simulink model "Identif_OpenLoop"  (R2023b)
settings: Solver=VariableStepAuto  StartTime=0.0  StopTime=80  FixedStep=0.0001  RelTol=1e-3
values from neighbouring files (symbols this model uses):
  C_T = Tg_ss / (r_r^4 * rho_air * pi * w_ss^2 * L_rod)    (= 0.0178337228008)    [model_constants.m]
  g = 9.81    [ArisonaIden.m]    (also in may13.m; model_constants.m = 9.806)
  J = 0.048    [ArisonaIden.m]    (also in may13.m; model_constants.m = 0.0161112)
  K_bldc = 131.3016804    [model_constants.m]
  K_f1 = r_r^4 * rho_air * pi * C_T    (= 5.49430535846e-06)    [model_constants.m]
  K_f2 = K_f1 * w_ss^2 / u_ss    (= 0.327888125)    [model_constants.m]
  L_g = (m_mot*L_rod + m_rod*L_rod/2)/(m_rod + m_mot)    (= 0.291818181818)    [model_constants.m]
  L_rod = 0.57    [ArisonaIden.m]    (also in model_constants.m = 0.42)
  m_mot = 0.06    [model_constants.m]
  m_rod = m_esc + m_ardu + m_wood    (= 0.094)    [model_constants.m]
  r_r = 0.095    [model_constants.m]
  rho_air = 1.204    [model_constants.m]
  Sample_Time = 0.025 * 2    (= 0.05)    [model_constants.m]
  T_bldc = 0.010214509    [model_constants.m]
undefined symbols (not defined in the file or in its folder): LF
libraries: slpidlib x8, instrumentseriallib x3, sldrtlib x2, svdutilitieslib x1
settings Model: SimulationMode=accelerator  Creator=Илья  LastModifiedBy=Илья

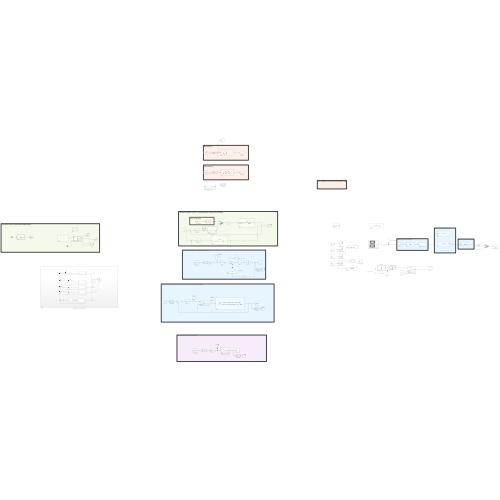
[thumbnail: Simulink's stored preview of the top-level diagram]
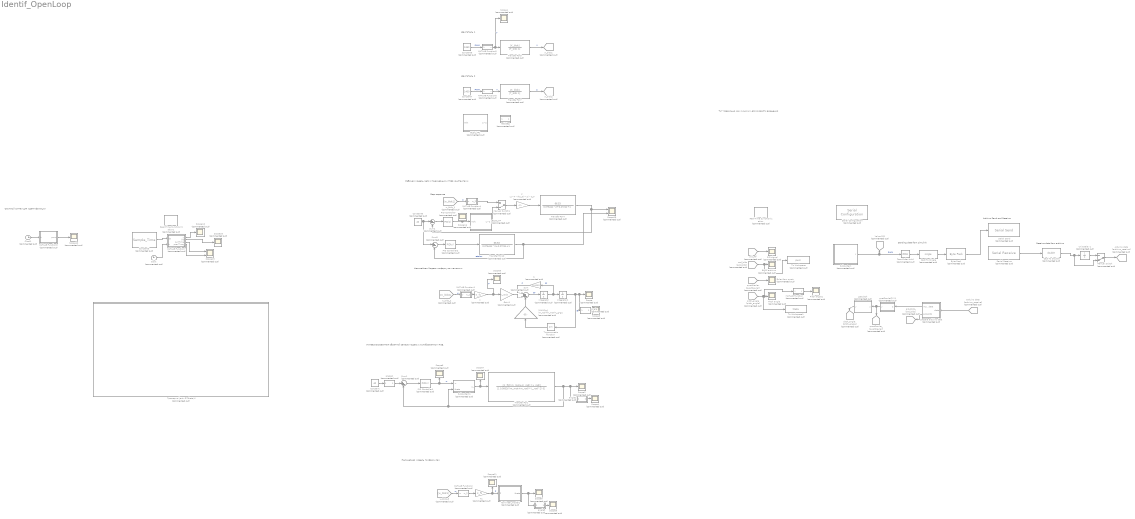
== system Identif_OpenLoop ==
  note: Нелинейная Модель из формулы механики
  note: Тут правильно как минимум для скорости вращения
  note: Sending data from simulink
  note: Arduino Send and Receive
  note: Receive data from arduino
  note: Step response
  note: Двигатель 1
  note: Двигатель 2
  note: Рабочая модель ijertv с подходящими ПИД константами
  note: Линеаризированная обратной связью модель с колиброванным ПИД
  note: Сложный сигнал для идентификации
  note: Нелинейная модель по формулам
  (M+M)lg/J : Gain  Commented=on  Gain=(m_rod+m_mot)*L_g*g/J
  Arduino data : Goto  Commented=on  GotoTag=arduino_receive
  BLDC arduino : Scope  Commented=on
  BLDC_TF : Subsystem  Commented=on
  BLDC_TF1 : Subsystem  Commented=on
  Byte Pack : svdutilitieslib/Byte Pack  Commented=on  maskPackedDataType=uint32  datatypes={'single'}  byteAlign=4  blockPlatform=arduinoert
  Cast To Double : DataTypeConversion  Commented=on  OutDataTypeStr=double  SaturateOnIntegerOverflow=off  RndMeth=Floor
  Cast To Single : DataTypeConversion  Commented=on  OutDataTypeStr=single  SaturateOnIntegerOverflow=off  RndMeth=Floor
  Clock : Clock  Commented=on
  Clock1 : Clock  Commented=on
  Constant : Constant  Commented=on  Value=40
  Constant3 : Constant  Commented=on  Value=Sample_Time
  Constant5 : Constant  Commented=on  Value=1350
  Constant6 : Constant  Commented=on  Value=40
  Constant7 : Constant  Commented=on  Value=1400
  Euler from quart : Scope  Commented=on
  F : Gain  Commented=on  Gain=r_r^4 * rho_air * pi * C_T
  Gain1 : Gain  Commented=on  Gain=L_rod/J
  Integrator : Integrator  Commented=on
  Integrator1 : Integrator  Commented=on
  K : Gain  Commented=on  Gain=K_f1
  K1 : Gain  Commented=on  Gain=K_f1
  MATLAB Function : MATLAB Function  Commented=on  TreatAsAtomicUnit=on
  MATLAB Function1 : MATLAB Function  Commented=on  TreatAsAtomicUnit=on
  MATLAB Function2 : MATLAB Function  Commented=on  TreatAsAtomicUnit=on
  MATLAB Function3 : MATLAB Function  Commented=on  TreatAsAtomicUnit=on
  MATLAB Function4 : MATLAB Function  Commented=on  TreatAsAtomicUnit=on
  MATLAB Function5 : MATLAB Function  Commented=on  TreatAsAtomicUnit=on
  MATLAB Function6 : MATLAB Function  Commented=on  TreatAsAtomicUnit=on
  MATLAB Function7 : MATLAB Function  Commented=on  TreatAsAtomicUnit=on  SystemSampleTime=Sample_Time
  Manual Switch : ManualSwitch  Commented=on  CurrentSetting=0
  Manual Switch1 : ManualSwitch  Commented=on  CurrentSetting=0
  Nonlinear_model1 : Subsystem  Commented=on
  PID Controller : slpidlib/PID Controller  Commented=on  Controller=PID  Form=Parallel  TimeDomain=Continuous-time  UseExternalTs=off  SampleTime=-1  IntegratorMethod=Forward Euler  FilterMethod=Forward Euler  ControllerParametersSource=internal  P=0.00834  I=0.0329  UseKiTs=off  D=0.00053  N=100  UseFilter=on  TunerSelectOption=Transfer Function Based (PID Tuner App)  InitialConditionSource=internal  InitialConditionForIntegrator=0  InitialConditionForFilter=0  DifferentiatorICPrevScaledInput=0  ExternalReset=none  TrackingMode=off  Kt=1  LimitOutput=off  SatLimitsSource=internal  UpperSaturationLimit=inf  LowerSaturationLimit=-inf  LinearizeAsGain=on  AntiWindupMode=none  Kb=1  LimitIntegrator=off  UpperIntegratorSaturationLimit=inf  LowerIntegratorSaturationLimit=-inf  POutMin=[]  POutMax=[]  IOutMin=[]  IOutMax=[]  DOutMin=[]  DOutMax=[]  NOutMin=[]  NOutMax=[]  SumOutMin=[]  SumOutMax=[]  SaturationOutMin=[]  SaturationOutMax=[]  PParamMin=[]  PParamMax=[]  IParamMin=[]  IParamMax=[]  DParamMin=[]  DParamMax=[]  NParamMin=[]  NParamMax=[]  KbParamMin=[]  KbParamMax=[]  KtParamMin=[]  KtParamMax=[]  KbOutMin=[]  KbOutMax=[]  KtOutMin=[]  KtOutMax=[]  IntegratorOutMin=[]  IntegratorOutMax=[]  FilterOutMin=[]  FilterOutMax=[]  SumI1OutMin=[]  SumI1OutMax=[]  SumI2OutMin=[]  SumI2OutMax=[]  SumI3OutMin=[]  SumI3OutMax=[]  SumI4OutMin=[]  SumI4OutMax=[]  SumDOutMin=[]  SumDOutMax=[]  DifferentiatorOutMin=[]  DifferentiatorOutMax=[]  FilterDiffOutCoefMin=[]  FilterDiffOutCoefMax=[]  ReciprocalOutMin=[]  ReciprocalOutMax=[]  SumDenOutMin=[]  SumDenOutMax=[]  SumNumOutMin=[]  SumNumOutMax=[]  DivideOutMin=[]  DivideOutMax=[]  UdiffTsProdOutMin=[]  UdiffTsProdOutMax=[]  NTsProdOutMin=[]  NTsProdOutMax=[]  UintegralTsProdOutMin=[]  UintegralTsProdOutMax=[]  UngainTsProdOutMin=[]  UngainTsProdOutMax=[]  ClampingZeroOutDataTypeStr=Inherit: Inherit via back propagation  ClampingZeroOutMin=[]  ClampingZeroOutMax=[]  FilterDenConstantOutDataTypeStr=Inherit: Inherit via back propagation  FilterDenConstantOutMin=[]  FilterDenConstantOutMax=[]  PCopyOutDataTypeStr=Inherit: Inherit via back propagation  PCopyOutMin=[]  PCopyOutMax=[]  NCopyOutDataTypeStr=Inherit: Inherit via back propagation  NCopyOutMin=[]  NCopyOutMax=[]  IntegratorContinuousStateAttributes=''  IntegratorStateMustResolveToSignalObject=off  IntegratorRTWStateStorageClass=Auto  FilterContinuousStateAttributes=''  FilterStateMustResolveToSignalObject=off  FilterRTWStateStorageClass=Auto  ParallelPVariant=InternalParameters  IdealPVariant=Disabled  IVariant=InternalParameters  DVariant=InternalParameters  IntegratorVariant=Continuous  SatVariant=Disabled  AWVariant=Passthrough  PCopyVariant=Disabled  TRVariant=Disabled  FdbkBlocksVariant=Forward  IdealPFdbkVariant=Disabled  SatFdbkVariant=Disabled  DerivativeFilterVariant=ContFilter  NVariant=InternalParameters  NCopyVariant=Disabled  FilterICVariant=InternalICsFilter  IntegratorICVariant=InternalICs  ExternalResetVariant=Disabled  TRSumVariant=Passthrough  SumFdbkVariant=Disabled  SumVariant=Sum_PID  TsampFilterVariant=InternalTs  TsampNgainVariant=Passthrough  TsampIntegralVariant=Disabled_SignalSpec  ExternalSaturationOutDataTypeStr=Inherit: Same as second input
  PID Controller1 : slpidlib/PID Controller  Commented=on  Controller=PID  Form=Parallel  TimeDomain=Continuous-time  UseExternalTs=off  SampleTime=-1  IntegratorMethod=Forward Euler  FilterMethod=Forward Euler  ControllerParametersSource=internal  P=822.969764124437  I=5665.62260200918  UseKiTs=off  D=29.2943119385291  N=827.781411873675  UseFilter=on  TunerSelectOption=Transfer Function Based (PID Tuner App)  InitialConditionSource=internal  InitialConditionForIntegrator=0  InitialConditionForFilter=0  DifferentiatorICPrevScaledInput=0  ExternalReset=none  TrackingMode=off  Kt=1  LimitOutput=off  SatLimitsSource=internal  UpperSaturationLimit=inf  LowerSaturationLimit=-inf  LinearizeAsGain=on  AntiWindupMode=none  Kb=1  LimitIntegrator=off  UpperIntegratorSaturationLimit=inf  LowerIntegratorSaturationLimit=-inf  POutMin=[]  POutMax=[]  IOutMin=[]  IOutMax=[]  DOutMin=[]  DOutMax=[]  NOutMin=[]  NOutMax=[]  SumOutMin=[]  SumOutMax=[]  SaturationOutMin=[]  SaturationOutMax=[]  PParamMin=[]  PParamMax=[]  IParamMin=[]  IParamMax=[]  DParamMin=[]  DParamMax=[]  NParamMin=[]  NParamMax=[]  KbParamMin=[]  KbParamMax=[]  KtParamMin=[]  KtParamMax=[]  KbOutMin=[]  KbOutMax=[]  KtOutMin=[]  KtOutMax=[]  IntegratorOutMin=[]  IntegratorOutMax=[]  FilterOutMin=[]  FilterOutMax=[]  SumI1OutMin=[]  SumI1OutMax=[]  SumI2OutMin=[]  SumI2OutMax=[]  SumI3OutMin=[]  SumI3OutMax=[]  SumI4OutMin=[]  SumI4OutMax=[]  SumDOutMin=[]  SumDOutMax=[]  DifferentiatorOutMin=[]  DifferentiatorOutMax=[]  FilterDiffOutCoefMin=[]  FilterDiffOutCoefMax=[]  ReciprocalOutMin=[]  ReciprocalOutMax=[]  SumDenOutMin=[]  SumDenOutMax=[]  SumNumOutMin=[]  SumNumOutMax=[]  DivideOutMin=[]  DivideOutMax=[]  UdiffTsProdOutMin=[]  UdiffTsProdOutMax=[]  NTsProdOutMin=[]  NTsProdOutMax=[]  UintegralTsProdOutMin=[]  UintegralTsProdOutMax=[]  UngainTsProdOutMin=[]  UngainTsProdOutMax=[]  ClampingZeroOutDataTypeStr=Inherit: Inherit via back propagation  ClampingZeroOutMin=[]  ClampingZeroOutMax=[]  FilterDenConstantOutDataTypeStr=Inherit: Inherit via back propagation  FilterDenConstantOutMin=[]  FilterDenConstantOutMax=[]  PCopyOutDataTypeStr=Inherit: Inherit via back propagation  PCopyOutMin=[]  PCopyOutMax=[]  NCopyOutDataTypeStr=Inherit: Inherit via back propagation  NCopyOutMin=[]  NCopyOutMax=[]  IntegratorContinuousStateAttributes=''  IntegratorStateMustResolveToSignalObject=off  IntegratorRTWStateStorageClass=Auto  FilterContinuousStateAttributes=''  FilterStateMustResolveToSignalObject=off  FilterRTWStateStorageClass=Auto  ParallelPVariant=InternalParameters  IdealPVariant=Disabled  IVariant=InternalParameters  DVariant=InternalParameters  IntegratorVariant=Continuous  SatVariant=Disabled  AWVariant=Passthrough  PCopyVariant=Disabled  TRVariant=Disabled  FdbkBlocksVariant=Forward  IdealPFdbkVariant=Disabled  SatFdbkVariant=Disabled  DerivativeFilterVariant=ContFilter  NVariant=InternalParameters  NCopyVariant=Disabled  FilterICVariant=InternalICsFilter  IntegratorICVariant=InternalICs  ExternalResetVariant=Disabled  TRSumVariant=Passthrough  SumFdbkVariant=Disabled  SumVariant=Sum_PID  TsampFilterVariant=InternalTs  TsampNgainVariant=Passthrough  TsampIntegralVariant=Disabled_SignalSpec  ExternalSaturationOutDataTypeStr=Inherit: Same as second input
  PID Controller2 : slpidlib/PID Controller  Commented=on  Controller=PID  Form=Parallel  TimeDomain=Continuous-time  UseExternalTs=off  SampleTime=-1  IntegratorMethod=Forward Euler  FilterMethod=Forward Euler  ControllerParametersSource=internal  P=0.00834  I=0.0329  UseKiTs=off  D=0.00053  N=100  UseFilter=on  TunerSelectOption=Transfer Function Based (PID Tuner App)  InitialConditionSource=internal  InitialConditionForIntegrator=0  InitialConditionForFilter=0  DifferentiatorICPrevScaledInput=0  ExternalReset=none  TrackingMode=off  Kt=1  LimitOutput=off  SatLimitsSource=internal  UpperSaturationLimit=inf  LowerSaturationLimit=-inf  LinearizeAsGain=on  AntiWindupMode=none  Kb=1  LimitIntegrator=off  UpperIntegratorSaturationLimit=inf  LowerIntegratorSaturationLimit=-inf  POutMin=[]  POutMax=[]  IOutMin=[]  IOutMax=[]  DOutMin=[]  DOutMax=[]  NOutMin=[]  NOutMax=[]  SumOutMin=[]  SumOutMax=[]  SaturationOutMin=[]  SaturationOutMax=[]  PParamMin=[]  PParamMax=[]  IParamMin=[]  IParamMax=[]  DParamMin=[]  DParamMax=[]  NParamMin=[]  NParamMax=[]  KbParamMin=[]  KbParamMax=[]  KtParamMin=[]  KtParamMax=[]  KbOutMin=[]  KbOutMax=[]  KtOutMin=[]  KtOutMax=[]  IntegratorOutMin=[]  IntegratorOutMax=[]  FilterOutMin=[]  FilterOutMax=[]  SumI1OutMin=[]  SumI1OutMax=[]  SumI2OutMin=[]  SumI2OutMax=[]  SumI3OutMin=[]  SumI3OutMax=[]  SumI4OutMin=[]  SumI4OutMax=[]  SumDOutMin=[]  SumDOutMax=[]  DifferentiatorOutMin=[]  DifferentiatorOutMax=[]  FilterDiffOutCoefMin=[]  FilterDiffOutCoefMax=[]  ReciprocalOutMin=[]  ReciprocalOutMax=[]  SumDenOutMin=[]  SumDenOutMax=[]  SumNumOutMin=[]  SumNumOutMax=[]  DivideOutMin=[]  DivideOutMax=[]  UdiffTsProdOutMin=[]  UdiffTsProdOutMax=[]  NTsProdOutMin=[]  NTsProdOutMax=[]  UintegralTsProdOutMin=[]  UintegralTsProdOutMax=[]  UngainTsProdOutMin=[]  UngainTsProdOutMax=[]  ClampingZeroOutDataTypeStr=Inherit: Inherit via back propagation  ClampingZeroOutMin=[]  ClampingZeroOutMax=[]  FilterDenConstantOutDataTypeStr=Inherit: Inherit via back propagation  FilterDenConstantOutMin=[]  FilterDenConstantOutMax=[]  PCopyOutDataTypeStr=Inherit: Inherit via back propagation  PCopyOutMin=[]  PCopyOutMax=[]  NCopyOutDataTypeStr=Inherit: Inherit via back propagation  NCopyOutMin=[]  NCopyOutMax=[]  IntegratorContinuousStateAttributes=''  IntegratorStateMustResolveToSignalObject=off  IntegratorRTWStateStorageClass=Auto  FilterContinuousStateAttributes=''  FilterStateMustResolveToSignalObject=off  FilterRTWStateStorageClass=Auto  ParallelPVariant=InternalParameters  IdealPVariant=Disabled  IVariant=InternalParameters  DVariant=InternalParameters  IntegratorVariant=Continuous  SatVariant=Disabled  AWVariant=Passthrough  PCopyVariant=Disabled  TRVariant=Disabled  FdbkBlocksVariant=Forward  IdealPFdbkVariant=Disabled  SatFdbkVariant=Disabled  DerivativeFilterVariant=ContFilter  NVariant=InternalParameters  NCopyVariant=Disabled  FilterICVariant=InternalICsFilter  IntegratorICVariant=InternalICs  ExternalResetVariant=Disabled  TRSumVariant=Passthrough  SumFdbkVariant=Disabled  SumVariant=Sum_PID  TsampFilterVariant=InternalTs  TsampNgainVariant=Passthrough  TsampIntegralVariant=Disabled_SignalSpec  ExternalSaturationOutDataTypeStr=Inherit: Same as second input
  PID signal : Scope  Commented=on
  Pitch angle : Scope  Commented=on
  Pitch angle1 : Scope  Commented=on
  Real-Time Synchronization : sldrtlib/Real-Time Synchronization  Commented=on  SampleTime=Sample_Time  MaxMissedTicks=2000  ShowMissedTicks=on  YieldWhenWaiting=off
  Real-Time Synchronization1 : sldrtlib/Real-Time Synchronization  Commented=on  SampleTime=0.05  MaxMissedTicks=2000  ShowMissedTicks=on  YieldWhenWaiting=off
  Scope{,1..12,16,20} (15 alike) : Scope  Commented=on
  Scope15 : Scope  Commented=on  NumInputPorts=2
  Scope19 : Scope  Commented=on  NumInputPorts=2
  Serial Configuration : instrumentseriallib/Serial Configuration  Priority=-200000  Commented=on  PortSel=COM3  Port=COM3  ComPort=COM3  BaudRate=115200  DataBits=8  Parity=none  StopBits=1  ByteOrder=little-endian  FlowControl=none  Timeout=10  SimulateUsing=Interpreted execution  BlockInModel=on  aMode=1
  Serial Receive : instrumentseriallib/Serial Receive  Priority=1  Commented=on  PortSel=COM3  Port=COM3  ComPort=COM3  DataType=single  SaveDataType=uint8  ToggleHeader=on  Header='A'  ToggleTerminator=on  Terminator=LF ('\n')  CustomTerminator=[]  InputFormat=Column major  ToggleDataSize=on  DataSize=[1 5]  EnableBlockingMode=on  ActionDataUnavailable=Output last received value  ActionWhenDataUnavailable=Output last received value  CustomValue=0  SampleTime=Sample_Time  SimulateUsing=Interpreted execution  BlockInModel=on  aMode=1
  Serial Send : instrumentseriallib/Serial Send  Priority=1  Commented=on  PortSel=COM3  Port=COM3  ComPort=COM3  Header=[]  Terminator=<none>  CustomTerminator=[]  EnableBlockingMode=on  SimulateUsing=Interpreted execution  BlockInModel=on  aMode=1
  Subsystem : Subsystem  Commented=on
  Subsystem1 : Subsystem  Commented=on
  Sum : Sum  Commented=on  Inputs=|-+-
  Sum1 : Sum  Commented=on  Inputs=|+-
  Sum2 : Sum  Commented=on  Inputs=|+-
  Sum8 : Sum  Commented=on  Inputs=|+-
  To Workspace : ToWorkspace  Commented=on  VariableName=pwm  SaveFormat=Timeseries  SampleTime=-1
  To Workspace1 : ToWorkspace  Commented=on  VariableName=theta  SaveFormat=Timeseries  SampleTime=-1
  Transfer Fcn1 : TransferFcn  Commented=on  Numerator=[K_f2/((m_mot+m_rod) * L_rod)]  Denominator=[1 0.0003/((m_mot+m_rod) * L_rod^2) 0]
  Transfer Fcn10 : TransferFcn  Commented=on  Numerator=[66.53]  Denominator=[0.07641 0.2721 1]
  Transfer Fcn4 : TransferFcn  Commented=on  Numerator=[66.53]  Denominator=[0.07641 0.2721 1]
  Transfer Fcn5 : TransferFcn  Commented=on  Numerator=[K_bldc]  Denominator=[T_bldc 1]
  Transfer Fcn7 : TransferFcn  Commented=on  Numerator=[K_bldc]  Denominator=[T_bldc 1]
  Trigonometric Function : Trigonometry  Commented=on
  Unit Delay1 : UnitDelay  Commented=on  SampleTime=0.1  HasFrameUpgradeWarning=on
  Value PID : Goto  Commented=on  GotoTag=pid_ref
  Zero-Order Hold : ZeroOrderHold  Commented=on  SampleTime=Sample_Time
  angle : MATLAB Function  Commented=on  TreatAsAtomicUnit=on
  angle1 : MATLAB Function  Commented=on  TreatAsAtomicUnit=on
  angle2 : MATLAB Function  Commented=on  TreatAsAtomicUnit=on
  angle3 : MATLAB Function  Commented=on  TreatAsAtomicUnit=on
  ard_bldc : From  Commented=on  GotoTag=ard_bldc
  ard_bldc_ : Goto  Commented=on  GotoTag=ard_bldc
  arduino data : From  Commented=on  GotoTag=arduino_receive
  b : Gain  Commented=on  Gain=0.0003
  get pitch : MATLAB Function  Commented=on  TreatAsAtomicUnit=on
  pid_ref : From  Commented=on  GotoTag=pid_ref
  pitch_angle : From  Commented=on  GotoTag=pitch_angle
  pitch_angle_ : Goto  Commented=on  GotoTag=pitch_angle
  prepare arduino data : Subsystem  Commented=on
  quart2euler : From  Commented=on  GotoTag=quart2euler
  quart2euler_ : Goto  Commented=on  GotoTag=quart2euler
  quat2eulerZYX1 : MATLAB Function  Commented=on  TreatAsAtomicUnit=on
  rad2deg : MATLAB Function  Commented=on  TreatAsAtomicUnit=on
  w_bldc1 : Goto  Commented=on  GotoTag=w_bldc1
  w_bldc2 : Goto  Commented=on  GotoTag=w_bldc2
  w_bldc_1 : From  Commented=on  GotoTag=w_bldc1
  w_bldc_2 : From  Commented=on  GotoTag=w_bldc1
  w_bldc_3 : From  Commented=on  GotoTag=w_bldc1
  Проверка ijertv G=theta/U : Subsystem  Commented=on
  wires:
  Integrator/1 -> b/1, Integrator1/1  "θ'"
  Integrator1/1 -> Trigonometric Function/1, angle/1(rad_), Scope/1  "θ"
  Sum/1 -> Integrator/1  "θ''"
  Trigonometric Function/1 -> (M+M)lg/J/1
  (M+M)lg/J/1 -> Sum/3
  K/1 -> Scope5/1, Gain1/1  "F"
  Gain1/1 -> Sum/2
  angle/1(deg_) -> Scope3/1
  Byte Pack/1 -> Serial Send/1
  quat2eulerZYX1/1(y) -> quart2euler_/1, get pitch/1(u)
  Cast To Single/1 -> Byte Pack/1
  Serial Receive/1 -> Cast To Double/1
  arduino data/1 -> prepare arduino data/1(data)
  Subsystem/1(y) -> Zero-Order Hold/1, Value PID/1  "PWM"
  prepare arduino data/1(mpu_data) -> quat2eulerZYX1/1(q)
  Cast To Double/1 -> Manual Switch/2, Unit Delay1/1
  prepare arduino data/2(ard_bldc) -> ard_bldc_/1
  pitch_angle/1 -> To Workspace1/1, MATLAB Function/1(u), Pitch angle/1
  Zero-Order Hold/1 -> Cast To Single/1
  Unit Delay1/1 -> Manual Switch/1
  ard_bldc/1 -> To Workspace/1, BLDC arduino/1
  quart2euler/1 -> Euler from quart/1
  Manual Switch/1 -> Arduino data/1
  pid_ref/1 -> PID signal/1
  get pitch/1(y) -> pitch_angle_/1
  MATLAB Function1/1(w_2) -> K/1
  Transfer Fcn4/1 -> Sum2/2, Scope15/1
  F/1 -> Transfer Fcn4/1
  PID Controller/1 -> BLDC_TF/1(Volt), Scope16/1
  BLDC_TF/1(ω^2) -> Manual Switch1/2
  Sum2/1 -> PID Controller/1
  Constant6/1 -> Sum8/1, Sum2/1
  Constant5/1 -> MATLAB Function5/1(pwm)  "PWM"
  MATLAB Function5/1(v) -> Scope1/1, Transfer Fcn5/1  "V"
  Transfer Fcn7/1 -> w_bldc2/1  "ω"
  MATLAB Function6/1(v) -> Transfer Fcn7/1  "V"
  Constant7/1 -> MATLAB Function6/1(pwm)  "PWM"
  MATLAB Function4/1(w_2) -> Manual Switch1/1
  w_bldc_1/1 -> MATLAB Function4/1(w)  "ω"
  Manual Switch1/1 -> F/1
  w_bldc_2/1 -> MATLAB Function1/1(w)  "ω"
  Transfer Fcn5/1 -> w_bldc1/1  "V"
  Constant/1 -> angle2/1(rad_)
  PID Controller1/1 -> Scope6/1, Subsystem1/1(w)  "w"
  Sum1/1 -> PID Controller1/1
  Subsystem1/1(u_) -> Scope7/1, Transfer Fcn1/1
  Transfer Fcn1/1 -> Sum1/2, Subsystem1/2(theta), angle1/1(rad_), Scope2/1
  angle1/1(deg_) -> Scope4/1
  angle2/1(deg_) -> Sum1/1
  w_bldc_3/1 -> MATLAB Function2/1(w)  "ω"
  MATLAB Function2/1(w_2) -> K1/1
  K1/1 -> Scope11/1, Nonlinear_model1/1(F)  "F"
  angle3/1(deg_) -> Scope9/1
  Nonlinear_model1/1(theta) -> angle3/1(rad_), Scope8/1
  MATLAB Function/1(y) -> Pitch angle1/1
  b/1 -> Sum/1  "F"
  MATLAB Function7/1(y) -> Scope10/1
  Constant3/1 -> MATLAB Function7/1(dt)
  Clock/1 -> MATLAB Function7/2(t)
  MATLAB Function7/3(currTime) -> Scope19/1
  MATLAB Function7/4(prevTime_) -> Scope19/2
  MATLAB Function7/2(ind) -> Scope20/1
  PID Controller2/1 -> Transfer Fcn10/1
  Sum8/1 -> PID Controller2/1
  Transfer Fcn10/1 -> Sum8/2, Scope15/2  "etalon"
  Clock1/1 -> MATLAB Function3/1(t)
  MATLAB Function3/1(pwm) -> Scope12/1

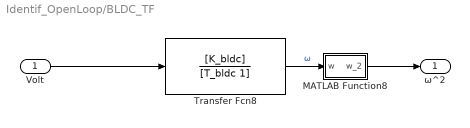
== system Identif_OpenLoop/BLDC_TF ==
  Volt : Inport
  MATLAB Function8 : MATLAB Function  TreatAsAtomicUnit=on
  Transfer Fcn8 : TransferFcn  Numerator=[K_bldc]  Denominator=[T_bldc 1]
  ω^2 : Outport
  wires:
  Transfer Fcn8/1 -> MATLAB Function8/1(w)  "ω"
  MATLAB Function8/1(w_2) -> ω^2/1
  Volt/1 -> Transfer Fcn8/1

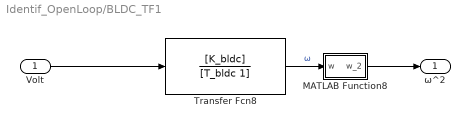
== system Identif_OpenLoop/BLDC_TF1 ==
  Volt : Inport
  MATLAB Function8 : MATLAB Function  TreatAsAtomicUnit=on
  Transfer Fcn8 : TransferFcn  Numerator=[K_bldc]  Denominator=[T_bldc 1]
  ω^2 : Outport
  wires:
  Volt/1 -> Transfer Fcn8/1
  MATLAB Function8/1(w_2) -> ω^2/1
  Transfer Fcn8/1 -> MATLAB Function8/1(w)  "ω"

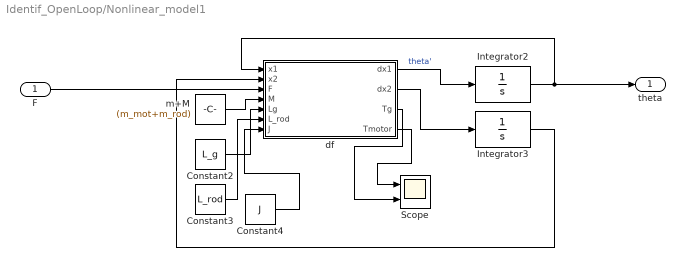
== system Identif_OpenLoop/Nonlinear_model1 ==
  F : Inport
  Constant2 : Constant  Value=L_g
  Constant3 : Constant  Value=L_rod
  Constant4 : Constant  Value=J
  Integrator2 : Integrator
  Integrator3 : Integrator
  Scope : Scope  NumInputPorts=2
  df : MATLAB Function  TreatAsAtomicUnit=on
  m+M : Constant  Value=(m_mot+m_rod)
  theta : Outport
  wires:
  df/1(dx1) -> Integrator2/1  "theta'"
  Integrator3/1 -> df/2(x2)
  Constant2/1 -> df/5(Lg)
  m+M/1 -> df/4(M)
  Constant4/1 -> df/7(J)
  Constant3/1 -> df/6(L_rod)
  Integrator2/1 -> df/1(x1), theta/1
  df/2(dx2) -> Integrator3/1
  F/1 -> df/3(F)
  df/4(Tmotor) -> Scope/1
  df/3(Tg) -> Scope/2

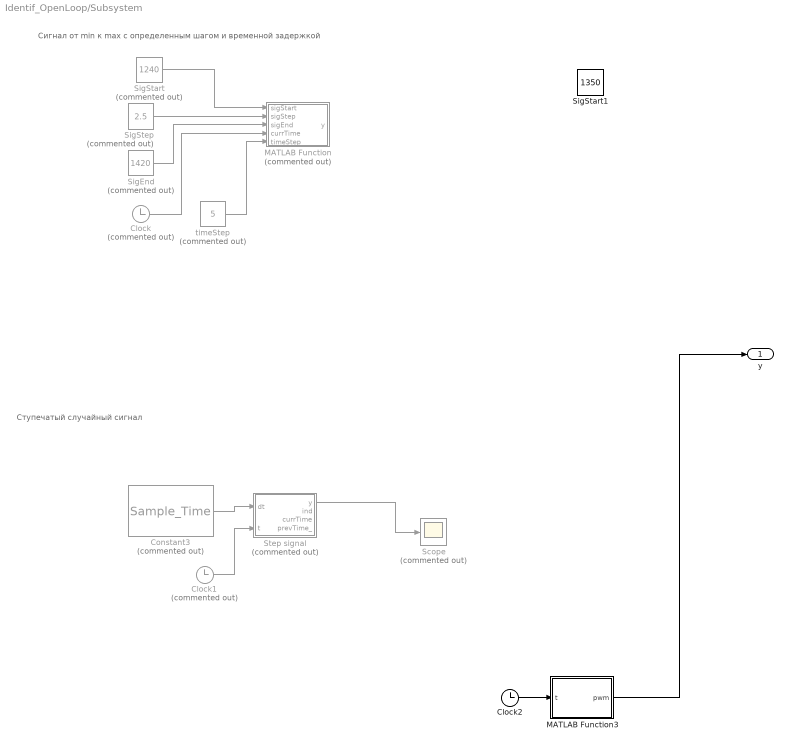
== system Identif_OpenLoop/Subsystem ==
  note: Сигнал от min к max с определенным шагом и временной задержкой
  note: Ступечатый случайный сигнал
  Clock : Clock  Commented=on
  Clock1 : Clock  Commented=on
  Clock2 : Clock
  Constant3 : Constant  Commented=on  Value=Sample_Time
  MATLAB Function : MATLAB Function  Commented=on  TreatAsAtomicUnit=on
  MATLAB Function3 : MATLAB Function  TreatAsAtomicUnit=on
  Scope : Scope  Commented=on
  SigEnd : Constant  Commented=on  Value=1420
  SigStart : Constant  Commented=on  Value=1240
  SigStart1 : Constant  Value=1350
  SigStep : Constant  Commented=on  Value=2.5
  Step signal : MATLAB Function  Commented=on  TreatAsAtomicUnit=on  SystemSampleTime=Sample_Time
  timeStep : Constant  Commented=on  Value=5
  y : Outport
  wires:
  SigStep/1 -> MATLAB Function/2(sigStep)
  SigEnd/1 -> MATLAB Function/3(sigEnd)
  SigStart/1 -> MATLAB Function/1(sigStart)
  Clock/1 -> MATLAB Function/4(currTime)
  timeStep/1 -> MATLAB Function/5(timeStep)
  Clock1/1 -> Step signal/2(t)
  Constant3/1 -> Step signal/1(dt)
  Step signal/1(y) -> Scope/1
  Clock2/1 -> MATLAB Function3/1(t)
  MATLAB Function3/1(pwm) -> y/1

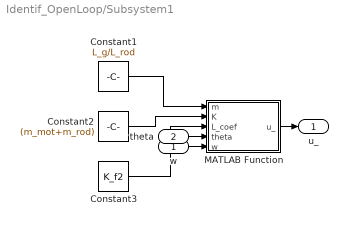
== system Identif_OpenLoop/Subsystem1 ==
  w : Inport
  theta : Inport  Port=2
  Constant1 : Constant  Value=L_g/L_rod
  Constant2 : Constant  Value=(m_mot+m_rod)
  Constant3 : Constant  Value=K_f2
  MATLAB Function : MATLAB Function  TreatAsAtomicUnit=on
  u_ : Outport
  wires:
  Constant3/1 -> MATLAB Function/3(L_coef)
  Constant1/1 -> MATLAB Function/1(m)
  w/1 -> MATLAB Function/5(w)
  Constant2/1 -> MATLAB Function/2(K)
  theta/1 -> MATLAB Function/4(theta)
  MATLAB Function/1(u_) -> u_/1

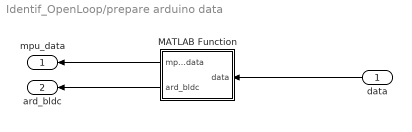
== system Identif_OpenLoop/prepare arduino data ==
  data : Inport
  MATLAB Function : MATLAB Function  TreatAsAtomicUnit=on
  mpu_data : Outport
  ard_bldc : Outport  Port=2
  wires:
  data/1 -> MATLAB Function/1(data)
  MATLAB Function/1(mpu_data) -> mpu_data/1
  MATLAB Function/2(ard_bldc) -> ard_bldc/1

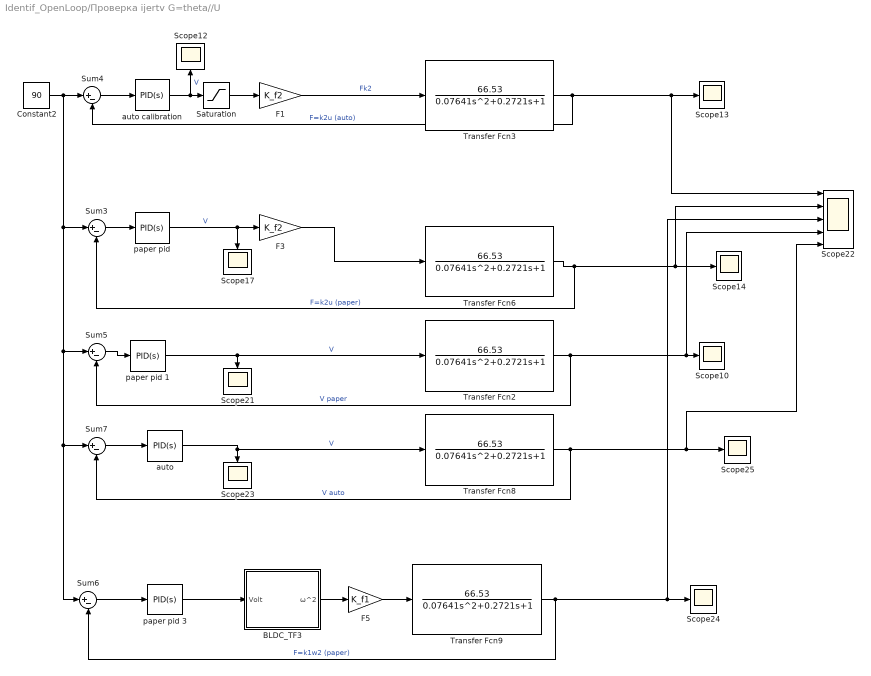
== system Identif_OpenLoop/Проверка ijertv G=theta//U ==
  BLDC_TF3 : Subsystem
  Constant2 : Constant  Value=90
  F1 : Gain  Gain=K_f2
  F3 : Gain  Gain=K_f2
  F5 : Gain  Gain=K_f1
  Saturation : Saturate  UpperLimit=11.1  LowerLimit=0
  Scope{10,12..14,17,21,23..25} (9 alike) : Scope
  Scope22 : Scope  NumInputPorts=5
  Sum{3..7} (5 alike) : Sum  Inputs=|+-
  Transfer Fcn{2..3,6,8..9} (5 alike) : TransferFcn  Numerator=[66.53]  Denominator=[0.07641 0.2721 1]
  auto : slpidlib/PID Controller  Controller=PID  Form=Parallel  TimeDomain=Continuous-time  UseExternalTs=off  SampleTime=-1  IntegratorMethod=Forward Euler  FilterMethod=Forward Euler  ControllerParametersSource=internal  P=0.398997891303364  I=0.900318180959032  UseKiTs=off  D=0.039580260390393  N=378.906023361119  UseFilter=on  TunerSelectOption=Transfer Function Based (PID Tuner App)  InitialConditionSource=internal  InitialConditionForIntegrator=0  InitialConditionForFilter=0  DifferentiatorICPrevScaledInput=0  ExternalReset=none  TrackingMode=off  Kt=1  LimitOutput=off  SatLimitsSource=internal  UpperSaturationLimit=inf  LowerSaturationLimit=-inf  LinearizeAsGain=on  AntiWindupMode=none  Kb=1  LimitIntegrator=off  UpperIntegratorSaturationLimit=inf  LowerIntegratorSaturationLimit=-inf  POutMin=[]  POutMax=[]  IOutMin=[]  IOutMax=[]  DOutMin=[]  DOutMax=[]  NOutMin=[]  NOutMax=[]  SumOutMin=[]  SumOutMax=[]  SaturationOutMin=[]  SaturationOutMax=[]  PParamMin=[]  PParamMax=[]  IParamMin=[]  IParamMax=[]  DParamMin=[]  DParamMax=[]  NParamMin=[]  NParamMax=[]  KbParamMin=[]  KbParamMax=[]  KtParamMin=[]  KtParamMax=[]  KbOutMin=[]  KbOutMax=[]  KtOutMin=[]  KtOutMax=[]  IntegratorOutMin=[]  IntegratorOutMax=[]  FilterOutMin=[]  FilterOutMax=[]  SumI1OutMin=[]  SumI1OutMax=[]  SumI2OutMin=[]  SumI2OutMax=[]  SumI3OutMin=[]  SumI3OutMax=[]  SumI4OutMin=[]  SumI4OutMax=[]  SumDOutMin=[]  SumDOutMax=[]  DifferentiatorOutMin=[]  DifferentiatorOutMax=[]  FilterDiffOutCoefMin=[]  FilterDiffOutCoefMax=[]  ReciprocalOutMin=[]  ReciprocalOutMax=[]  SumDenOutMin=[]  SumDenOutMax=[]  SumNumOutMin=[]  SumNumOutMax=[]  DivideOutMin=[]  DivideOutMax=[]  UdiffTsProdOutMin=[]  UdiffTsProdOutMax=[]  NTsProdOutMin=[]  NTsProdOutMax=[]  UintegralTsProdOutMin=[]  UintegralTsProdOutMax=[]  UngainTsProdOutMin=[]  UngainTsProdOutMax=[]  ClampingZeroOutDataTypeStr=Inherit: Inherit via back propagation  ClampingZeroOutMin=[]  ClampingZeroOutMax=[]  FilterDenConstantOutDataTypeStr=Inherit: Inherit via back propagation  FilterDenConstantOutMin=[]  FilterDenConstantOutMax=[]  PCopyOutDataTypeStr=Inherit: Inherit via back propagation  PCopyOutMin=[]  PCopyOutMax=[]  NCopyOutDataTypeStr=Inherit: Inherit via back propagation  NCopyOutMin=[]  NCopyOutMax=[]  IntegratorContinuousStateAttributes=''  IntegratorStateMustResolveToSignalObject=off  IntegratorRTWStateStorageClass=Auto  FilterContinuousStateAttributes=''  FilterStateMustResolveToSignalObject=off  FilterRTWStateStorageClass=Auto  ParallelPVariant=InternalParameters  IdealPVariant=Disabled  IVariant=InternalParameters  DVariant=InternalParameters  IntegratorVariant=Continuous  SatVariant=Disabled  AWVariant=Passthrough  PCopyVariant=Disabled  TRVariant=Disabled  FdbkBlocksVariant=Forward  IdealPFdbkVariant=Disabled  SatFdbkVariant=Disabled  DerivativeFilterVariant=ContFilter  NVariant=InternalParameters  NCopyVariant=Disabled  FilterICVariant=InternalICsFilter  IntegratorICVariant=InternalICs  ExternalResetVariant=Disabled  TRSumVariant=Passthrough  SumFdbkVariant=Disabled  SumVariant=Sum_PID  TsampFilterVariant=InternalTs  TsampNgainVariant=Passthrough  TsampIntegralVariant=Disabled_SignalSpec  ExternalSaturationOutDataTypeStr=Inherit: Same as second input
  auto calibration : slpidlib/PID Controller  Controller=PID  Form=Parallel  TimeDomain=Continuous-time  UseExternalTs=off  SampleTime=-1  IntegratorMethod=Forward Euler  FilterMethod=Forward Euler  ControllerParametersSource=internal  P=1.61298683383668  I=4.55996186415523  UseKiTs=off  D=0.128826815470178  N=144.438379913464  UseFilter=on  TunerSelectOption=Transfer Function Based (PID Tuner App)  InitialConditionSource=internal  InitialConditionForIntegrator=0  InitialConditionForFilter=0  DifferentiatorICPrevScaledInput=0  ExternalReset=none  TrackingMode=off  Kt=1  LimitOutput=off  SatLimitsSource=internal  UpperSaturationLimit=inf  LowerSaturationLimit=-inf  LinearizeAsGain=on  AntiWindupMode=none  Kb=1  LimitIntegrator=off  UpperIntegratorSaturationLimit=inf  LowerIntegratorSaturationLimit=-inf  POutMin=[]  POutMax=[]  IOutMin=[]  IOutMax=[]  DOutMin=[]  DOutMax=[]  NOutMin=[]  NOutMax=[]  SumOutMin=[]  SumOutMax=[]  SaturationOutMin=[]  SaturationOutMax=[]  PParamMin=[]  PParamMax=[]  IParamMin=[]  IParamMax=[]  DParamMin=[]  DParamMax=[]  NParamMin=[]  NParamMax=[]  KbParamMin=[]  KbParamMax=[]  KtParamMin=[]  KtParamMax=[]  KbOutMin=[]  KbOutMax=[]  KtOutMin=[]  KtOutMax=[]  IntegratorOutMin=[]  IntegratorOutMax=[]  FilterOutMin=[]  FilterOutMax=[]  SumI1OutMin=[]  SumI1OutMax=[]  SumI2OutMin=[]  SumI2OutMax=[]  SumI3OutMin=[]  SumI3OutMax=[]  SumI4OutMin=[]  SumI4OutMax=[]  SumDOutMin=[]  SumDOutMax=[]  DifferentiatorOutMin=[]  DifferentiatorOutMax=[]  FilterDiffOutCoefMin=[]  FilterDiffOutCoefMax=[]  ReciprocalOutMin=[]  ReciprocalOutMax=[]  SumDenOutMin=[]  SumDenOutMax=[]  SumNumOutMin=[]  SumNumOutMax=[]  DivideOutMin=[]  DivideOutMax=[]  UdiffTsProdOutMin=[]  UdiffTsProdOutMax=[]  NTsProdOutMin=[]  NTsProdOutMax=[]  UintegralTsProdOutMin=[]  UintegralTsProdOutMax=[]  UngainTsProdOutMin=[]  UngainTsProdOutMax=[]  ClampingZeroOutDataTypeStr=Inherit: Inherit via back propagation  ClampingZeroOutMin=[]  ClampingZeroOutMax=[]  FilterDenConstantOutDataTypeStr=Inherit: Inherit via back propagation  FilterDenConstantOutMin=[]  FilterDenConstantOutMax=[]  PCopyOutDataTypeStr=Inherit: Inherit via back propagation  PCopyOutMin=[]  PCopyOutMax=[]  NCopyOutDataTypeStr=Inherit: Inherit via back propagation  NCopyOutMin=[]  NCopyOutMax=[]  IntegratorContinuousStateAttributes=''  IntegratorStateMustResolveToSignalObject=off  IntegratorRTWStateStorageClass=Auto  FilterContinuousStateAttributes=''  FilterStateMustResolveToSignalObject=off  FilterRTWStateStorageClass=Auto  ParallelPVariant=InternalParameters  IdealPVariant=Disabled  IVariant=InternalParameters  DVariant=InternalParameters  IntegratorVariant=Continuous  SatVariant=Disabled  AWVariant=Passthrough  PCopyVariant=Disabled  TRVariant=Disabled  FdbkBlocksVariant=Forward  IdealPFdbkVariant=Disabled  SatFdbkVariant=Disabled  DerivativeFilterVariant=ContFilter  NVariant=InternalParameters  NCopyVariant=Disabled  FilterICVariant=InternalICsFilter  IntegratorICVariant=InternalICs  ExternalResetVariant=Disabled  TRSumVariant=Passthrough  SumFdbkVariant=Disabled  SumVariant=Sum_PID  TsampFilterVariant=InternalTs  TsampNgainVariant=Passthrough  TsampIntegralVariant=Disabled_SignalSpec  ExternalSaturationOutDataTypeStr=Inherit: Same as second input
  paper pid : slpidlib/PID Controller  Controller=PID  Form=Parallel  TimeDomain=Continuous-time  UseExternalTs=off  SampleTime=-1  IntegratorMethod=Forward Euler  FilterMethod=Forward Euler  ControllerParametersSource=internal  P=0.00834  I=0.0329  UseKiTs=off  D=0.00053  N=100  UseFilter=on  TunerSelectOption=Transfer Function Based (PID Tuner App)  InitialConditionSource=internal  InitialConditionForIntegrator=0  InitialConditionForFilter=0  DifferentiatorICPrevScaledInput=0  ExternalReset=none  TrackingMode=off  Kt=1  LimitOutput=off  SatLimitsSource=internal  UpperSaturationLimit=inf  LowerSaturationLimit=-inf  LinearizeAsGain=on  AntiWindupMode=none  Kb=1  LimitIntegrator=off  UpperIntegratorSaturationLimit=inf  LowerIntegratorSaturationLimit=-inf  POutMin=[]  POutMax=[]  IOutMin=[]  IOutMax=[]  DOutMin=[]  DOutMax=[]  NOutMin=[]  NOutMax=[]  SumOutMin=[]  SumOutMax=[]  SaturationOutMin=[]  SaturationOutMax=[]  PParamMin=[]  PParamMax=[]  IParamMin=[]  IParamMax=[]  DParamMin=[]  DParamMax=[]  NParamMin=[]  NParamMax=[]  KbParamMin=[]  KbParamMax=[]  KtParamMin=[]  KtParamMax=[]  KbOutMin=[]  KbOutMax=[]  KtOutMin=[]  KtOutMax=[]  IntegratorOutMin=[]  IntegratorOutMax=[]  FilterOutMin=[]  FilterOutMax=[]  SumI1OutMin=[]  SumI1OutMax=[]  SumI2OutMin=[]  SumI2OutMax=[]  SumI3OutMin=[]  SumI3OutMax=[]  SumI4OutMin=[]  SumI4OutMax=[]  SumDOutMin=[]  SumDOutMax=[]  DifferentiatorOutMin=[]  DifferentiatorOutMax=[]  FilterDiffOutCoefMin=[]  FilterDiffOutCoefMax=[]  ReciprocalOutMin=[]  ReciprocalOutMax=[]  SumDenOutMin=[]  SumDenOutMax=[]  SumNumOutMin=[]  SumNumOutMax=[]  DivideOutMin=[]  DivideOutMax=[]  UdiffTsProdOutMin=[]  UdiffTsProdOutMax=[]  NTsProdOutMin=[]  NTsProdOutMax=[]  UintegralTsProdOutMin=[]  UintegralTsProdOutMax=[]  UngainTsProdOutMin=[]  UngainTsProdOutMax=[]  ClampingZeroOutDataTypeStr=Inherit: Inherit via back propagation  ClampingZeroOutMin=[]  ClampingZeroOutMax=[]  FilterDenConstantOutDataTypeStr=Inherit: Inherit via back propagation  FilterDenConstantOutMin=[]  FilterDenConstantOutMax=[]  PCopyOutDataTypeStr=Inherit: Inherit via back propagation  PCopyOutMin=[]  PCopyOutMax=[]  NCopyOutDataTypeStr=Inherit: Inherit via back propagation  NCopyOutMin=[]  NCopyOutMax=[]  IntegratorContinuousStateAttributes=''  IntegratorStateMustResolveToSignalObject=off  IntegratorRTWStateStorageClass=Auto  FilterContinuousStateAttributes=''  FilterStateMustResolveToSignalObject=off  FilterRTWStateStorageClass=Auto  ParallelPVariant=InternalParameters  IdealPVariant=Disabled  IVariant=InternalParameters  DVariant=InternalParameters  IntegratorVariant=Continuous  SatVariant=Disabled  AWVariant=Passthrough  PCopyVariant=Disabled  TRVariant=Disabled  FdbkBlocksVariant=Forward  IdealPFdbkVariant=Disabled  SatFdbkVariant=Disabled  DerivativeFilterVariant=ContFilter  NVariant=InternalParameters  NCopyVariant=Disabled  FilterICVariant=InternalICsFilter  IntegratorICVariant=InternalICs  ExternalResetVariant=Disabled  TRSumVariant=Passthrough  SumFdbkVariant=Disabled  SumVariant=Sum_PID  TsampFilterVariant=InternalTs  TsampNgainVariant=Passthrough  TsampIntegralVariant=Disabled_SignalSpec  ExternalSaturationOutDataTypeStr=Inherit: Same as second input
  paper pid 1 : slpidlib/PID Controller  Controller=PID  Form=Parallel  TimeDomain=Continuous-time  UseExternalTs=off  SampleTime=-1  IntegratorMethod=Forward Euler  FilterMethod=Forward Euler  ControllerParametersSource=internal  P=0.00834  I=0.0329  UseKiTs=off  D=0.00053  N=100  UseFilter=on  TunerSelectOption=Transfer Function Based (PID Tuner App)  InitialConditionSource=internal  InitialConditionForIntegrator=0  InitialConditionForFilter=0  DifferentiatorICPrevScaledInput=0  ExternalReset=none  TrackingMode=off  Kt=1  LimitOutput=off  SatLimitsSource=internal  UpperSaturationLimit=inf  LowerSaturationLimit=-inf  LinearizeAsGain=on  AntiWindupMode=none  Kb=1  LimitIntegrator=off  UpperIntegratorSaturationLimit=inf  LowerIntegratorSaturationLimit=-inf  POutMin=[]  POutMax=[]  IOutMin=[]  IOutMax=[]  DOutMin=[]  DOutMax=[]  NOutMin=[]  NOutMax=[]  SumOutMin=[]  SumOutMax=[]  SaturationOutMin=[]  SaturationOutMax=[]  PParamMin=[]  PParamMax=[]  IParamMin=[]  IParamMax=[]  DParamMin=[]  DParamMax=[]  NParamMin=[]  NParamMax=[]  KbParamMin=[]  KbParamMax=[]  KtParamMin=[]  KtParamMax=[]  KbOutMin=[]  KbOutMax=[]  KtOutMin=[]  KtOutMax=[]  IntegratorOutMin=[]  IntegratorOutMax=[]  FilterOutMin=[]  FilterOutMax=[]  SumI1OutMin=[]  SumI1OutMax=[]  SumI2OutMin=[]  SumI2OutMax=[]  SumI3OutMin=[]  SumI3OutMax=[]  SumI4OutMin=[]  SumI4OutMax=[]  SumDOutMin=[]  SumDOutMax=[]  DifferentiatorOutMin=[]  DifferentiatorOutMax=[]  FilterDiffOutCoefMin=[]  FilterDiffOutCoefMax=[]  ReciprocalOutMin=[]  ReciprocalOutMax=[]  SumDenOutMin=[]  SumDenOutMax=[]  SumNumOutMin=[]  SumNumOutMax=[]  DivideOutMin=[]  DivideOutMax=[]  UdiffTsProdOutMin=[]  UdiffTsProdOutMax=[]  NTsProdOutMin=[]  NTsProdOutMax=[]  UintegralTsProdOutMin=[]  UintegralTsProdOutMax=[]  UngainTsProdOutMin=[]  UngainTsProdOutMax=[]  ClampingZeroOutDataTypeStr=Inherit: Inherit via back propagation  ClampingZeroOutMin=[]  ClampingZeroOutMax=[]  FilterDenConstantOutDataTypeStr=Inherit: Inherit via back propagation  FilterDenConstantOutMin=[]  FilterDenConstantOutMax=[]  PCopyOutDataTypeStr=Inherit: Inherit via back propagation  PCopyOutMin=[]  PCopyOutMax=[]  NCopyOutDataTypeStr=Inherit: Inherit via back propagation  NCopyOutMin=[]  NCopyOutMax=[]  IntegratorContinuousStateAttributes=''  IntegratorStateMustResolveToSignalObject=off  IntegratorRTWStateStorageClass=Auto  FilterContinuousStateAttributes=''  FilterStateMustResolveToSignalObject=off  FilterRTWStateStorageClass=Auto  ParallelPVariant=InternalParameters  IdealPVariant=Disabled  IVariant=InternalParameters  DVariant=InternalParameters  IntegratorVariant=Continuous  SatVariant=Disabled  AWVariant=Passthrough  PCopyVariant=Disabled  TRVariant=Disabled  FdbkBlocksVariant=Forward  IdealPFdbkVariant=Disabled  SatFdbkVariant=Disabled  DerivativeFilterVariant=ContFilter  NVariant=InternalParameters  NCopyVariant=Disabled  FilterICVariant=InternalICsFilter  IntegratorICVariant=InternalICs  ExternalResetVariant=Disabled  TRSumVariant=Passthrough  SumFdbkVariant=Disabled  SumVariant=Sum_PID  TsampFilterVariant=InternalTs  TsampNgainVariant=Passthrough  TsampIntegralVariant=Disabled_SignalSpec  ExternalSaturationOutDataTypeStr=Inherit: Same as second input
  paper pid 3 : slpidlib/PID Controller  Controller=PID  Form=Parallel  TimeDomain=Continuous-time  UseExternalTs=off  SampleTime=-1  IntegratorMethod=Forward Euler  FilterMethod=Forward Euler  ControllerParametersSource=internal  P=0.00834  I=0.0329  UseKiTs=off  D=0.00053  N=100  UseFilter=on  TunerSelectOption=Transfer Function Based (PID Tuner App)  InitialConditionSource=internal  InitialConditionForIntegrator=0  InitialConditionForFilter=0  DifferentiatorICPrevScaledInput=0  ExternalReset=none  TrackingMode=off  Kt=1  LimitOutput=off  SatLimitsSource=internal  UpperSaturationLimit=inf  LowerSaturationLimit=-inf  LinearizeAsGain=on  AntiWindupMode=none  Kb=1  LimitIntegrator=off  UpperIntegratorSaturationLimit=inf  LowerIntegratorSaturationLimit=-inf  POutMin=[]  POutMax=[]  IOutMin=[]  IOutMax=[]  DOutMin=[]  DOutMax=[]  NOutMin=[]  NOutMax=[]  SumOutMin=[]  SumOutMax=[]  SaturationOutMin=[]  SaturationOutMax=[]  PParamMin=[]  PParamMax=[]  IParamMin=[]  IParamMax=[]  DParamMin=[]  DParamMax=[]  NParamMin=[]  NParamMax=[]  KbParamMin=[]  KbParamMax=[]  KtParamMin=[]  KtParamMax=[]  KbOutMin=[]  KbOutMax=[]  KtOutMin=[]  KtOutMax=[]  IntegratorOutMin=[]  IntegratorOutMax=[]  FilterOutMin=[]  FilterOutMax=[]  SumI1OutMin=[]  SumI1OutMax=[]  SumI2OutMin=[]  SumI2OutMax=[]  SumI3OutMin=[]  SumI3OutMax=[]  SumI4OutMin=[]  SumI4OutMax=[]  SumDOutMin=[]  SumDOutMax=[]  DifferentiatorOutMin=[]  DifferentiatorOutMax=[]  FilterDiffOutCoefMin=[]  FilterDiffOutCoefMax=[]  ReciprocalOutMin=[]  ReciprocalOutMax=[]  SumDenOutMin=[]  SumDenOutMax=[]  SumNumOutMin=[]  SumNumOutMax=[]  DivideOutMin=[]  DivideOutMax=[]  UdiffTsProdOutMin=[]  UdiffTsProdOutMax=[]  NTsProdOutMin=[]  NTsProdOutMax=[]  UintegralTsProdOutMin=[]  UintegralTsProdOutMax=[]  UngainTsProdOutMin=[]  UngainTsProdOutMax=[]  ClampingZeroOutDataTypeStr=Inherit: Inherit via back propagation  ClampingZeroOutMin=[]  ClampingZeroOutMax=[]  FilterDenConstantOutDataTypeStr=Inherit: Inherit via back propagation  FilterDenConstantOutMin=[]  FilterDenConstantOutMax=[]  PCopyOutDataTypeStr=Inherit: Inherit via back propagation  PCopyOutMin=[]  PCopyOutMax=[]  NCopyOutDataTypeStr=Inherit: Inherit via back propagation  NCopyOutMin=[]  NCopyOutMax=[]  IntegratorContinuousStateAttributes=''  IntegratorStateMustResolveToSignalObject=off  IntegratorRTWStateStorageClass=Auto  FilterContinuousStateAttributes=''  FilterStateMustResolveToSignalObject=off  FilterRTWStateStorageClass=Auto  ParallelPVariant=InternalParameters  IdealPVariant=Disabled  IVariant=InternalParameters  DVariant=InternalParameters  IntegratorVariant=Continuous  SatVariant=Disabled  AWVariant=Passthrough  PCopyVariant=Disabled  TRVariant=Disabled  FdbkBlocksVariant=Forward  IdealPFdbkVariant=Disabled  SatFdbkVariant=Disabled  DerivativeFilterVariant=ContFilter  NVariant=InternalParameters  NCopyVariant=Disabled  FilterICVariant=InternalICsFilter  IntegratorICVariant=InternalICs  ExternalResetVariant=Disabled  TRSumVariant=Passthrough  SumFdbkVariant=Disabled  SumVariant=Sum_PID  TsampFilterVariant=InternalTs  TsampNgainVariant=Passthrough  TsampIntegralVariant=Disabled_SignalSpec  ExternalSaturationOutDataTypeStr=Inherit: Same as second input
  wires:
  Sum3/1 -> paper pid/1
  Sum4/1 -> auto calibration/1
  F3/1 -> Transfer Fcn6/1
  auto calibration/1 -> Scope12/1, Saturation/1  "V"
  Transfer Fcn2/1 -> Sum5/2, Scope22/4, Scope10/1  "V paper"
  Transfer Fcn9/1 -> Sum6/2, Scope22/3, Scope24/1  "F=k1w2 (paper)"
  Transfer Fcn3/1 -> Sum4/2, Scope22/1, Scope13/1  "F=k2u (auto)"
  Transfer Fcn6/1 -> Sum3/2, Scope22/2, Scope14/1  "F=k2u (paper)"
  paper pid 3/1 -> BLDC_TF3/1(Volt)
  Sum6/1 -> paper pid 3/1
  Constant2/1 -> Sum7/1, Sum6/1, Sum5/1, Sum3/1, Sum4/1
  Transfer Fcn8/1 -> Scope22/5, Scope25/1, Sum7/2  "V auto"
  paper pid/1 -> Scope17/1, F3/1  "V"
  F1/1 -> Transfer Fcn3/1  "Fk2"
  paper pid 1/1 -> Scope21/1, Transfer Fcn2/1  "V"
  Saturation/1 -> F1/1
  Sum7/1 -> auto/1
  BLDC_TF3/1(ω^2) -> F5/1
  F5/1 -> Transfer Fcn9/1
  auto/1 -> Transfer Fcn8/1, Scope23/1  "V"
  Sum5/1 -> paper pid 1/1

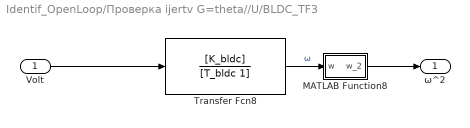
== system Identif_OpenLoop/Проверка ijertv G=theta//U/BLDC_TF3 ==
  Volt : Inport
  MATLAB Function8 : MATLAB Function  TreatAsAtomicUnit=on
  Transfer Fcn8 : TransferFcn  Numerator=[K_bldc]  Denominator=[T_bldc 1]
  ω^2 : Outport
  wires:
  Volt/1 -> Transfer Fcn8/1
  MATLAB Function8/1(w_2) -> ω^2/1
  Transfer Fcn8/1 -> MATLAB Function8/1(w)  "ω"

== matlab function Identif_OpenLoop/MATLAB Function4 ==
  data: w input; w_2 output
function w_2 = fcn(w)

w_2 = w^2;

== matlab function Identif_OpenLoop/MATLAB Function5 ==
  data: pwm input; v output
function v = fcn(pwm)
min_volt = 0;
max_volt = 11.1;

min_pwm = 1200;
max_pwm = 2000;

v = rescale(pwm, min_volt, max_volt, "InputMin", min_pwm, "InputMax", max_pwm);

== matlab function Identif_OpenLoop/MATLAB Function6 ==
  data: pwm input; v output
function v = fcn(pwm)
min_volt = 0;
max_volt = 11.1;

min_pwm = 1200;
max_pwm = 2000;

v = rescale(pwm, min_volt, max_volt, "InputMin", min_pwm, "InputMax", max_pwm);

== matlab function Identif_OpenLoop/BLDC_TF1/MATLAB Function8 ==
  data: w input; w_2 output
function w_2 = fcn(w)

w_2 = w^2;

== matlab function Identif_OpenLoop/BLDC_TF/MATLAB Function8 ==
  data: w input; w_2 output
function w_2 = fcn(w)

w_2 = w^2;

== matlab function Identif_OpenLoop/MATLAB Function2 ==
  data: w input; w_2 output
function w_2 = fcn(w)

w_2 = w^2;

== matlab function Identif_OpenLoop/angle3 ==
  data: rad_ input; deg_ output
function deg_ = fcn(rad_)

%deg_ = rad2deg(rad_);
deg_ = mod(rad2deg(rad_), 360);

== matlab function Identif_OpenLoop/Subsystem1/MATLAB Function ==
  data: m input; u_ output; K input; L_coef input; theta input; w input
function u_ = fcn(m, K, L_coef, theta, w)

u_ = m*9.81/K * sin(theta) * L_coef  + w;

== matlab function Identif_OpenLoop/MATLAB Function ==
  data: u input; y output
function y = fcn(u)

y = 90+u;

== matlab function Identif_OpenLoop/Subsystem/Step signal ==
  settings: updateMethod=DISCRETE
  data: dt input; y output; t input; ind output; currTime output; prevTime_ output
function [y, ind, currTime, prevTime_] = fcn(dt, t)
total_time = 80;

%rng("shuffle");
persistent pwm_arr
if isempty(pwm_arr)
    % time width
    time_width_arr = randi([1 3], total_time, 1);
    % get count of signals
    sum = 0;
    count_ind = 0;
    time_width_arr=time_width_arr(randperm(length(time_width_arr)));
    for i = 1:length(time_width_arr)
        sum = sum + time_width_arr(i);
        if sum > total_time
            count_ind = i;
            break;
        end
    end    
    tmp = 1240 + 180 * rand(count_ind,1);
    pwm_arr = [];
    %disp(time_width_arr)
   % disp(tmp)
    for i = 1:length(tmp)
        %fprintf("%d %f %d %d", i, tmp(i), time_width_arr(i), int32(time_width_arr(i) / dt));
        %disp([i, tmp(i), time_width_arr(i), int32(time_width_arr(i) / dt)]);
        pwm_arr = [pwm_arr, repelem(tmp(i), int32(time_width_arr(i) / dt))];
    end
end

persistent currInd
if isempty(currInd)
    currInd = 1;
end

persistent prevTime
if isempty(prevTime)
    prevTime = 0;
end

%if (t - prevTime) >= dt
if (t > prevTime)
    currInd = currInd + 1;
    prevTime = t;
end
y = pwm_arr(currInd);
currTime = t;
prevTime_ = prevTime;
ind = currInd;

== matlab function Identif_OpenLoop/MATLAB Function7 ==
  settings: updateMethod=DISCRETE
  data: dt input; y output; t input; ind output; currTime output; prevTime_ output
function [y, ind, currTime, prevTime_] = fcn(dt, t)
total_time = 80;

%rng("shuffle");
persistent pwm_arr
if isempty(pwm_arr)
    % time width
    time_width_arr = randi([1 2], total_time, 1);
    % get count of signals
    sum = 0;
    count_ind = 0;
    time_width_arr=time_width_arr(randperm(length(time_width_arr)));
    for i = 1:length(time_width_arr)
        sum = sum + time_width_arr(i);
        if sum > total_time
            count_ind = i;
            break;
        end
    end    
    tmp = 1240 + 180 * rand(count_ind,1);
    pwm_arr = [];
    disp(time_width_arr)
    disp(tmp)
    for i = 1:length(tmp)
        %fprintf("%d %f %d %d", i, tmp(i), time_width_arr(i), int32(time_width_arr(i) / dt));
        disp([i, tmp(i), time_width_arr(i), int32(time_width_arr(i) / dt)]);
        pwm_arr = [pwm_arr, repelem(tmp(i), int32(time_width_arr(i) / dt))];
    end
end

persistent currInd
if isempty(currInd)
    currInd = 1;
end

persistent prevTime
if isempty(prevTime)
    prevTime = 0;
end

%if (t - prevTime) >= dt
if (t > prevTime)
    currInd = currInd + 1;
    prevTime = t;
end
y = pwm_arr(currInd);
currTime = t;
prevTime_ = prevTime;
ind = currInd;

== matlab function Identif_OpenLoop/MATLAB Function3 ==
  data: t input; pwm output
function pwm = fcn(t)

add_min = 1260;
add_dop = 78+5;

a0 = 13;
a1 = 2.5;
a2 = 4;
a3 = 2;

b1 = 1;
b2 = 0.4;
b3 = 0.1;


pwm = add_min + add_dop + a0*(a1*sin(b1*t) + a2 * cos(b2 * t + 4) + a3 * sin(b3*t));

== matlab function Identif_OpenLoop/Subsystem/MATLAB Function3 ==
  data: t input; pwm output
function pwm = fcn(t)

add_min = 1260;
add_dop = 78 - 1;

a0 = 12 + 1;
a1 = 2.5;
a2 = 4;
a3 = 2;

b1 = 1;
b2 = 0.4;
b3 = 0.1;


%pwm = add_min + add_dop + a0*(a1*sin(b1*t) + a2 * cos(b2 * t + 4) + a3 * sin(b3*t));
% alter signal for test
pwm = 1260 + 90 + 12 * (2.4 * sin(1.1*t) + 4 * cos(0.6*t + 3) + 2 * sin(1.5*t + 1));

== matlab function Identif_OpenLoop/Проверка ijertv G=theta//U/BLDC_TF3/MATLAB Function8 ==
  data: w input; w_2 output
function w_2 = fcn(w)

w_2 = w^2;

== matlab function Identif_OpenLoop/angle ==
  data: rad_ input; deg_ output
function deg_ = fcn(rad_)

%deg_ = rad2deg(rad_);
deg_ = mod(rad2deg(rad_), 360);

== matlab function Identif_OpenLoop/Subsystem/MATLAB Function ==
  settings: updateMethod=DISCRETE
  data: y output; sigStart input; sigStep input; sigEnd input; currTime input; timeStep input
function y = fcn(sigStart, sigStep, sigEnd, currTime, timeStep)

persistent constArray;
if isempty(constArray)
    constArray = sigStart:sigStep:sigEnd;
end

persistent timeMemory;
if isempty(timeMemory)
    timeMemory = 0;
end

persistent index;
if isempty(index)
    index = 1;
end


if ((currTime - timeMemory) >= timeStep)
    index = index + 1;
    if (index > length(constArray))
        index = length(constArray);
    end
    timeMemory = timeMemory + timeStep;
    disp(constArray(index));
end



y = constArray(index);

== matlab function Identif_OpenLoop/angle2 ==
  data: rad_ input; deg_ output
function deg_ = fcn(rad_)

%deg_ = rad2deg(rad_);
deg_ = deg2rad(rad_);

== matlab function Identif_OpenLoop/quat2eulerZYX1 ==
  data: q input; y output
function y = fcn(q)

y = rad2deg(quat2eul(q, "ZYX"));

== matlab function Identif_OpenLoop/get pitch ==
  data: u input; y output
function y = fcn(u)
% 3
y = u(2);

== matlab function Identif_OpenLoop/prepare arduino data/MATLAB Function ==
  data: data input; mpu_data output; ard_bldc output
function [mpu_data , ard_bldc] = fcn(data)
mpu_data = data(1:end-1);
ard_bldc = data(end);

== matlab function Identif_OpenLoop/MATLAB Function1 ==
  data: w input; w_2 output
function w_2 = fcn(w)

w_2 = w^2;

== matlab function Identif_OpenLoop/rad2deg ==
  data: rad_ input; deg_ output
function deg_ = fcn(rad_)

deg_ =mod(rad2deg(rad_), 360);

== matlab function Identif_OpenLoop/angle1 ==
  data: rad_ input; deg_ output
function deg_ = fcn(rad_)

%deg_ = rad2deg(rad_);
deg_ = mod(rad2deg(rad_), 360);

== matlab function Identif_OpenLoop/Nonlinear_model1/df ==
  data: x1 input; x2 input; F input; dx1 output; dx2 output; M input; Lg input; L_rod input; J input; Tg output; Tmotor output
function [dx1, dx2, Tg, Tmotor] = fcn(x1, x2, F, M, Lg, L_rod, J)
% x1 = theta
% x2 = theta'

dx1 = x2;
dx2 = -M*9.81*Lg*sin(x1)/J - 0.006*x2/J + L_rod*F/J;
%dx2 = -M*9.81*Lg*sin(x1)/J + L_rod*F/J;
Tg = -M*9.81*Lg*sin(x1)/J;
Tmotor = L_rod*F/J;
